simulink model "sys1"  (R2015a)
settings: Solver=ode45  StartTime=0.0  StopTime=1000  RelTol=1e-3
values from neighbouring files (symbols this model uses):
  sys = ss(A,B,C,D)    [ABCD.m]
settings Model: Creator=Ivan  LastModifiedBy=Ivan

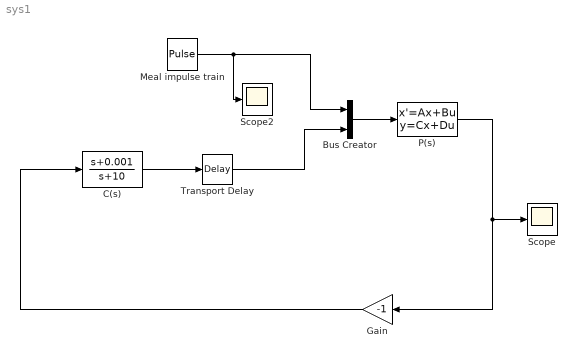
== system sys1 ==
  Bus Creator : BusCreator  Inputs=2
  C(s) : TransferFcn  Numerator=[1 0.001]  Denominator=[1 10]
  Gain : Gain  Gain=-1
  Meal impulse train : DiscretePulseGenerator  PulseType=Time based  Amplitude=10  Period=400  PulseWidth=0.001
  P(s) : StateSpace  A=sys.A  B=sys.B  C=sys.C  D=sys.D  X0=0
  Scope : Scope
      settings: TimeRange=1000  YMin=0  YMax=0.2
  Scope2 : Scope
      settings: SaveName=ScopeData2
  Transport Delay : TransportDelay  DelayTime=100
  wires:
  Gain/1 -> C(s)/1
  Meal impulse train/1 -> Bus Creator/1, Scope2/1
  P(s)/1 -> Gain/1, Scope/1
  C(s)/1 -> Transport Delay/1
  Transport Delay/1 -> Bus Creator/2
  Bus Creator/1 -> P(s)/1
